simulink model "HighLevelPlatform"  (R2018b)
settings: Solver=VariableStepAuto  StartTime=0.0  StopTime=tsim  FixedStep=tstep  RelTol=1e-3
values from neighbouring files (symbols this model uses):
  tsim = 10    [Platform.m]
settings Model: Creator=Erin B  LastModifiedBy=embeato2
settings SolverCC: ZeroCrossAlgorithm=Adaptive
settings DebuggingCC: IgnoredZcDiagnostic=none

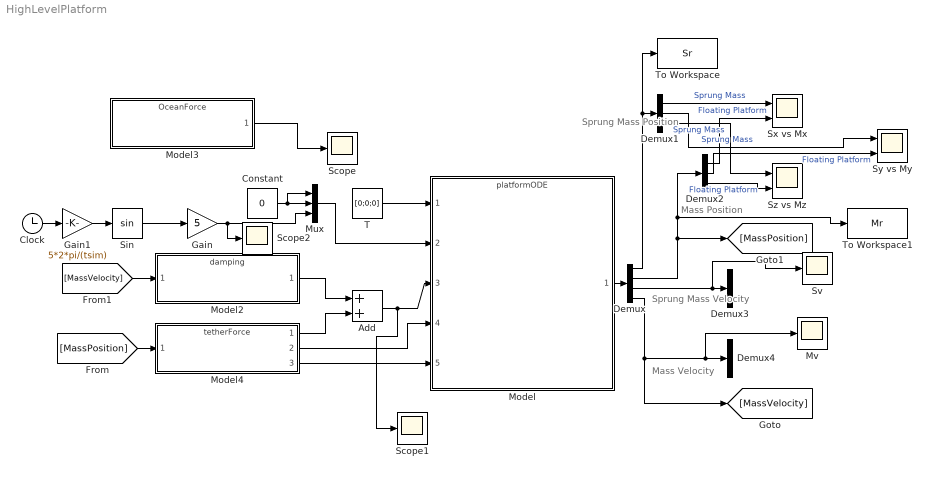
== system HighLevelPlatform ==
  note: Mass Velocity
  note: Sprung Mass Velocity
  note: Mass Position
  note: Sprung Mass Position
  Add : Sum
  Clock : Clock
  Constant : Constant  Value=0
  Demux : Demux
  Demux{1..4} (4 alike) : Demux  Outputs=3
  Gain : Gain  Gain=5
  Gain1 : Gain  Gain=5*2*pi/(tsim)
  Model : ModelReference  ModelNameDialog=platformODE  SimulationMode=Normal  ModelReferenceVersion=1.33
  Model2 : ModelReference  ModelNameDialog=damping.slx  SimulationMode=Normal  ModelReferenceVersion=1.6
  Model3 : ModelReference  ModelNameDialog=OceanForce.slx  SimulationMode=Normal  ModelReferenceVersion=1.4
  Model4 : ModelReference  ModelNameDialog=tetherForce  SimulationMode=Normal  ModelReferenceVersion=1.4
  Mux : Mux  Inputs=3
  Mv : Scope
  Scope : Scope
  Scope1 : Scope
  Scope2 : Scope
  Sin : Trigonometry
  Sv : Scope
  Sx vs Mx : Scope  NumInputPorts=2
  Sy vs My : Scope  NumInputPorts=2
  Sz vs Mz : Scope  NumInputPorts=2
  T : Constant  Value=[0;0;0]
  To Workspace : ToWorkspace  VariableName=Sr  SaveFormat=Timeseries  SampleTime=-1
  To Workspace1 : ToWorkspace  VariableName=Mr  SaveFormat=Timeseries  SampleTime=-1
  wires:
  Demux/1 -> To Workspace/1, Demux1/1
  Demux/2 -> [MassPosition], To Workspace1/1, Demux2/1
  Demux/3 -> Sv/1, Demux3/1
  Demux/4 -> [MassVelocity], Mv/1, Demux4/1
  Demux1/3 -> Sz vs Mz/1  "Sprung Mass"
  Demux2/3 -> Sz vs Mz/2  "Floating Platform"
  Model/1 -> Demux/1
  Demux2/1 -> Sx vs Mx/2  "Floating Platform"
  T/1 -> Model/1
  Constant/1 -> Mux/1, Mux/2
  Mux/1 -> Model/2
  Add/1 -> Scope1/1, Model/3
  Demux1/1 -> Sx vs Mx/1  "Sprung Mass"
  [MassVelocity] -> Model2/1
  Demux2/2 -> Sy vs My/2  "Floating Platform"
  Demux1/2 -> Sy vs My/1  "Sprung Mass"
  Model3/1 -> Scope/1
  [MassPosition] -> Model4/1
  Model4/1 -> Add/2
  Model4/2 -> Model/4
  Model4/3 -> Model/5
  Model2/1 -> Add/1
  Clock/1 -> Gain1/1
  Sin/1 -> Gain/1
  Gain/1 -> Scope2/1, Mux/3
  Gain1/1 -> Sin/1
